simulink model "Final_Q2_j"  (R2019a)
settings: Solver=ode1  StartTime=0.0  StopTime=60  FixedStep=0.01  RelTol=1e-3  EnableMultiTasking=on
libraries: simulink x4
settings Model: Creator=enesu  LastModifiedBy=hp
settings SolverCC: AutoInsertRateTranBlk=on

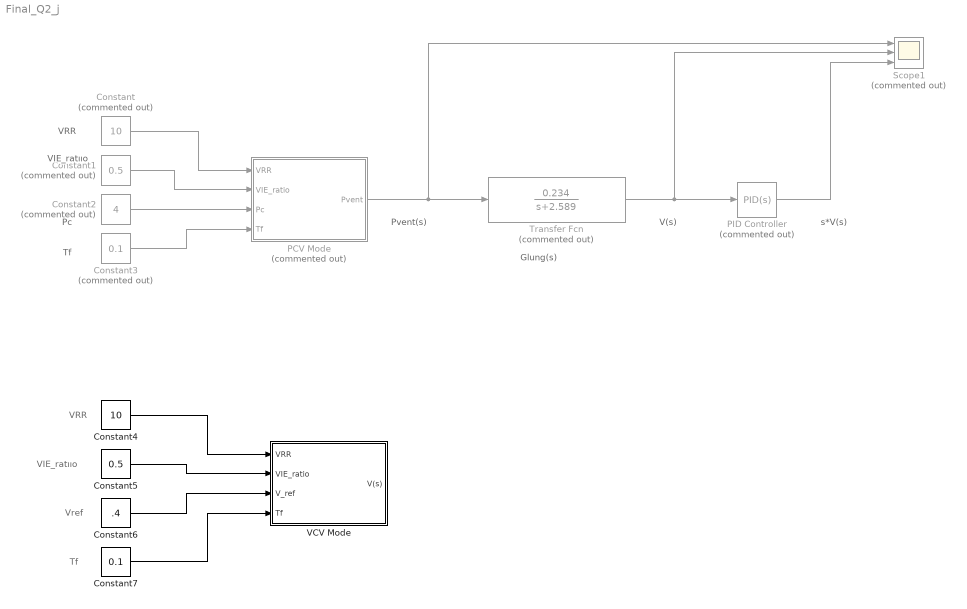
== system Final_Q2_j ==
  note: VIE_ratııo
  note: VRR
  note: Tf
  note: Vref
  note: VIE_ratııo
  note: VRR
  note: Pvent(s)
  note: Glung(s)
  note: s*V(s)
  note: V(s)
  note: Pc
  note: Tf
  Constant : Constant  Commented=on  Value=10  VectorParams1D=off
  Constant1 : Constant  Commented=on  Value=0.5
  Constant2 : Constant  Commented=on  Value=4
  Constant3 : Constant  Commented=on  Value=0.1
  Constant4 : Constant  Value=10
  Constant5 : Constant  Value=0.5
  Constant6 : Constant  Value=.4
  Constant7 : Constant  Value=0.1
  PCV Mode : Subsystem  Commented=on
  PID Controller : simulink/Continuous/PID Controller  Commented=on  Controller=PID  Form=Parallel  TimeDomain=Continuous-time  SampleTime=-1  IntegratorMethod=Forward Euler  FilterMethod=Forward Euler  ControllerParametersSource=internal  P=0  I=0  D=1  UseFilter=on  N=100  TunerSelectOption=Transfer Function Based (PID Tuner App)  InitialConditionSource=internal  InitialConditionForIntegrator=0  InitialConditionForFilter=0  DifferentiatorICPrevScaledInput=0  ExternalReset=none  TrackingMode=off  Kt=1  LimitOutput=off  UpperSaturationLimit=inf  LowerSaturationLimit=-inf  LinearizeAsGain=on  AntiWindupMode=none  Kb=1  POutMin=[]  POutMax=[]  IOutMin=[]  IOutMax=[]  DOutMin=[]  DOutMax=[]  NOutMin=[]  NOutMax=[]  SumOutMin=[]  SumOutMax=[]  SaturationOutMin=[]  SaturationOutMax=[]  PParamMin=[]  PParamMax=[]  IParamMin=[]  IParamMax=[]  DParamMin=[]  DParamMax=[]  NParamMin=[]  NParamMax=[]  KbParamMin=[]  KbParamMax=[]  KtParamMin=[]  KtParamMax=[]  KbOutMin=[]  KbOutMax=[]  KtOutMin=[]  KtOutMax=[]  IntegratorOutMin=[]  IntegratorOutMax=[]  FilterOutMin=[]  FilterOutMax=[]  SumI1OutMin=[]  SumI1OutMax=[]  SumI2OutMin=[]  SumI2OutMax=[]  SumI3OutMin=[]  SumI3OutMax=[]  SumI4OutMin=[]  SumI4OutMax=[]  SumDOutMin=[]  SumDOutMax=[]  DifferentiatorOutMin=[]  DifferentiatorOutMax=[]  FilterDiffOutCoefMin=[]  FilterDiffOutCoefMax=[]  ReciprocalOutMin=[]  ReciprocalOutMax=[]  SumDenOutMin=[]  SumDenOutMax=[]  SumNumOutMin=[]  SumNumOutMax=[]  DivideOutMin=[]  DivideOutMax=[]  IntegratorContinuousStateAttributes=''  IntegratorStateMustResolveToSignalObject=off  IntegratorRTWStateStorageClass=Auto  FilterContinuousStateAttributes=''  FilterStateMustResolveToSignalObject=off  FilterRTWStateStorageClass=Auto  ParallelPVariant=InternalParameters  IdealPVariant=Disabled  IVariant=InternalParameters  DVariant=InternalParameters  IntegratorVariant=Continuous  SatVariant=Disabled  AWVariant=Passthrough  PCopyVariant=Disabled  TRVariant=Disabled  FdbkBlocksVariant=Forward  IdealPFdbkVariant=Disabled  SatFdbkVariant=Disabled  DerivativeFilterVariant=ContFilter  NVariant=InternalParameters  NCopyVariant=Disabled  FilterICVariant=InternalICsFilter  IntegratorICVariant=InternalICs  ExternalResetVariant=Disabled  TRSumVariant=Passthrough  SumFdbkVariant=Disabled  SumVariant=Sum_PID
  Scope1 : Scope  Commented=on  NumInputPorts=3
  Transfer Fcn : TransferFcn  Commented=on  Numerator=[ 0.234 ]  Denominator=[1 2.589]
  VCV Mode : Subsystem
  wires:
  Constant/1 -> PCV Mode/1(VRR)
  Constant1/1 -> PCV Mode/2(VIE_ratio)
  Constant2/1 -> PCV Mode/3(Pc)
  Transfer Fcn/1 -> Scope1/2, PID Controller/1
  Constant3/1 -> PCV Mode/4(Tf)
  Constant6/1 -> VCV Mode/3(V_ref)
  Constant5/1 -> VCV Mode/2(VIE_ratio)
  Constant4/1 -> VCV Mode/1(VRR)
  PID Controller/1 -> Scope1/3
  Constant7/1 -> VCV Mode/4(Tf)
  PCV Mode/1(Pvent) -> Scope1/1, Transfer Fcn/1

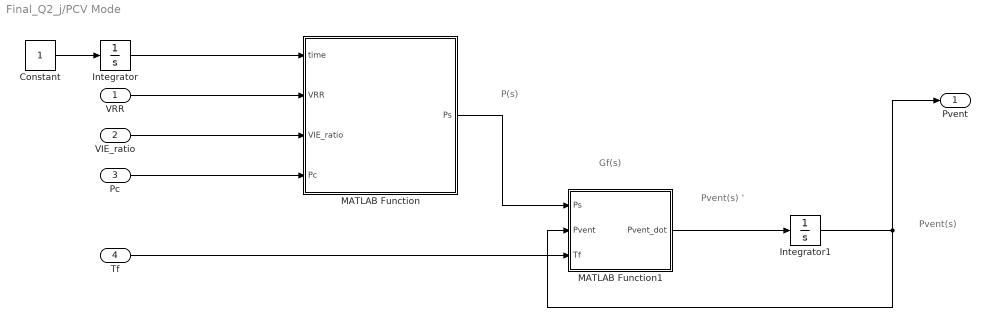
== system Final_Q2_j/PCV Mode ==
  note: P(s)
  note: Gf(s)
  note: Pvent(s) '
  note: Pvent(s)
  VRR : Inport
  VIE_ratio : Inport  Port=2
  Pc : Inport  Port=3
  Tf : Inport  Port=4
  Constant : Constant
  Integrator : Integrator
  Integrator1 : Integrator
  MATLAB Function : MATLAB Function  TreatAsAtomicUnit=on
  MATLAB Function1 : MATLAB Function  TreatAsAtomicUnit=on
  Pvent : Outport  VectorParamsAs1DForOutWhenUnconnected=on
  wires:
  Constant/1 -> Integrator/1
  Integrator/1 -> MATLAB Function/1(time)
  VRR/1 -> MATLAB Function/2(VRR)
  VIE_ratio/1 -> MATLAB Function/3(VIE_ratio)
  Pc/1 -> MATLAB Function/4(Pc)
  Tf/1 -> MATLAB Function1/3(Tf)
  MATLAB Function/1(Ps) -> MATLAB Function1/1(Ps)
  MATLAB Function1/1(Pvent_dot) -> Integrator1/1
  Integrator1/1 -> Pvent/1, MATLAB Function1/2(Pvent)

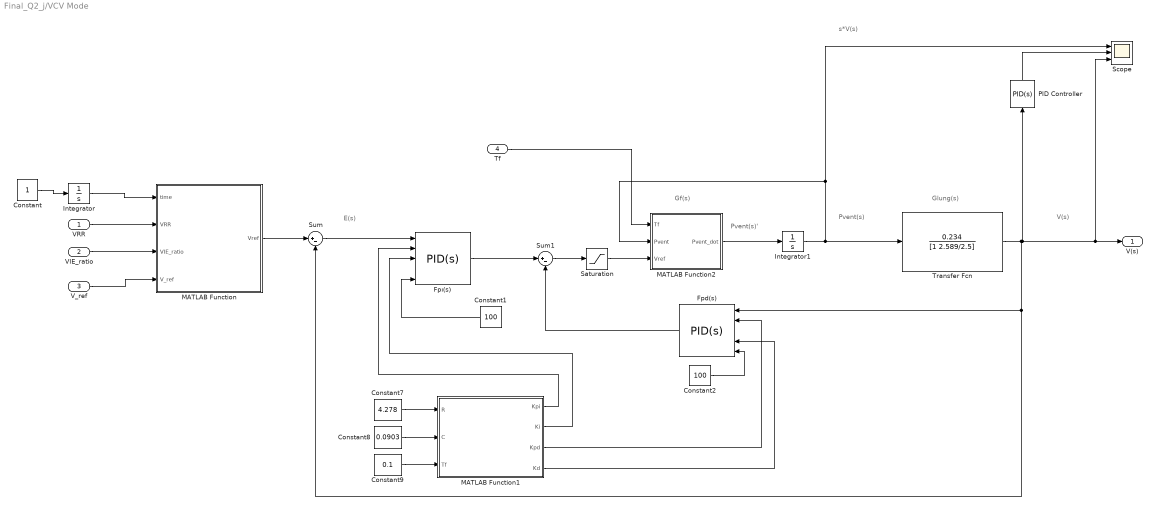
== system Final_Q2_j/VCV Mode ==
  note: Gf(s)
  note: Glung(s)
  note: s*V(s)
  note: V(s)
  note: Pvent(s)'
  note: Pvent(s)
  note: E(s)
  VRR : Inport
  VIE_ratio : Inport  Port=2
  V_ref : Inport  Port=3
  Tf : Inport  Port=4
  Constant : Constant
  Constant1 : Constant  Value=100
  Constant2 : Constant  Value=100
  Constant7 : Constant  Value=4.278
  Constant8 : Constant  Value=0.0903
  Constant9 : Constant  Value=0.1
  Fpd(s) : simulink/Continuous/PID Controller  Controller=PID  Form=Parallel  TimeDomain=Continuous-time  SampleTime=-1  IntegratorMethod=Forward Euler  FilterMethod=Forward Euler  ControllerParametersSource=external  P=1  I=1  D=0  UseFilter=on  N=100  TunerSelectOption=Transfer Function Based (PID Tuner App)  InitialConditionSource=internal  InitialConditionForIntegrator=0  InitialConditionForFilter=0  DifferentiatorICPrevScaledInput=0  ExternalReset=none  TrackingMode=off  Kt=1  LimitOutput=off  UpperSaturationLimit=115  LowerSaturationLimit=0  LinearizeAsGain=on  AntiWindupMode=none  Kb=1  POutMin=[]  POutMax=[]  IOutMin=[]  IOutMax=[]  DOutMin=[]  DOutMax=[]  NOutMin=[]  NOutMax=[]  SumOutMin=[]  SumOutMax=[]  SaturationOutMin=[]  SaturationOutMax=[]  PParamMin=[]  PParamMax=[]  IParamMin=[]  IParamMax=[]  DParamMin=[]  DParamMax=[]  NParamMin=[]  NParamMax=[]  KbParamMin=[]  KbParamMax=[]  KtParamMin=[]  KtParamMax=[]  KbOutMin=[]  KbOutMax=[]  KtOutMin=[]  KtOutMax=[]  IntegratorOutMin=[]  IntegratorOutMax=[]  FilterOutMin=[]  FilterOutMax=[]  SumI1OutMin=[]  SumI1OutMax=[]  SumI2OutMin=[]  SumI2OutMax=[]  SumI3OutMin=[]  SumI3OutMax=[]  SumI4OutMin=[]  SumI4OutMax=[]  SumDOutMin=[]  SumDOutMax=[]  DifferentiatorOutMin=[]  DifferentiatorOutMax=[]  FilterDiffOutCoefMin=[]  FilterDiffOutCoefMax=[]  ReciprocalOutMin=[]  ReciprocalOutMax=[]  SumDenOutMin=[]  SumDenOutMax=[]  SumNumOutMin=[]  SumNumOutMax=[]  DivideOutMin=[]  DivideOutMax=[]  IntegratorContinuousStateAttributes=''  IntegratorStateMustResolveToSignalObject=off  IntegratorRTWStateStorageClass=Auto  FilterContinuousStateAttributes=''  FilterStateMustResolveToSignalObject=off  FilterRTWStateStorageClass=Auto  ParallelPVariant=ExternalParameters  IdealPVariant=Disabled  IVariant=ExternalParameters  DVariant=ExternalParameters  IntegratorVariant=Continuous  SatVariant=Disabled  AWVariant=Passthrough  PCopyVariant=Disabled  TRVariant=Disabled  FdbkBlocksVariant=Forward  IdealPFdbkVariant=Disabled  SatFdbkVariant=Disabled  DerivativeFilterVariant=ContFilter  NVariant=ExternalParameters  NCopyVariant=Disabled  FilterICVariant=InternalICsFilter  IntegratorICVariant=InternalICs  ExternalResetVariant=Disabled  TRSumVariant=Passthrough  SumFdbkVariant=Disabled  SumVariant=Sum_PID
  Fpı(s) : simulink/Continuous/PID Controller  Controller=PID  Form=Parallel  TimeDomain=Continuous-time  SampleTime=-1  IntegratorMethod=Forward Euler  FilterMethod=Forward Euler  ControllerParametersSource=external  P=1  I=1  D=0  UseFilter=on  N=100  TunerSelectOption=Transfer Function Based (PID Tuner App)  InitialConditionSource=internal  InitialConditionForIntegrator=0  InitialConditionForFilter=0  DifferentiatorICPrevScaledInput=0  ExternalReset=none  TrackingMode=off  Kt=1  LimitOutput=off  UpperSaturationLimit=inf  LowerSaturationLimit=0  LinearizeAsGain=on  AntiWindupMode=none  Kb=1  POutMin=[]  POutMax=[]  IOutMin=[]  IOutMax=[]  DOutMin=[]  DOutMax=[]  NOutMin=[]  NOutMax=[]  SumOutMin=[]  SumOutMax=[]  SaturationOutMin=[]  SaturationOutMax=[]  PParamMin=[]  PParamMax=[]  IParamMin=[]  IParamMax=[]  DParamMin=[]  DParamMax=[]  NParamMin=[]  NParamMax=[]  KbParamMin=[]  KbParamMax=[]  KtParamMin=[]  KtParamMax=[]  KbOutMin=[]  KbOutMax=[]  KtOutMin=[]  KtOutMax=[]  IntegratorOutMin=[]  IntegratorOutMax=[]  FilterOutMin=[]  FilterOutMax=[]  SumI1OutMin=[]  SumI1OutMax=[]  SumI2OutMin=[]  SumI2OutMax=[]  SumI3OutMin=[]  SumI3OutMax=[]  SumI4OutMin=[]  SumI4OutMax=[]  SumDOutMin=[]  SumDOutMax=[]  DifferentiatorOutMin=[]  DifferentiatorOutMax=[]  FilterDiffOutCoefMin=[]  FilterDiffOutCoefMax=[]  ReciprocalOutMin=[]  ReciprocalOutMax=[]  SumDenOutMin=[]  SumDenOutMax=[]  SumNumOutMin=[]  SumNumOutMax=[]  DivideOutMin=[]  DivideOutMax=[]  IntegratorContinuousStateAttributes=''  IntegratorStateMustResolveToSignalObject=off  IntegratorRTWStateStorageClass=Auto  FilterContinuousStateAttributes=''  FilterStateMustResolveToSignalObject=off  FilterRTWStateStorageClass=Auto  ParallelPVariant=ExternalParameters  IdealPVariant=Disabled  IVariant=ExternalParameters  DVariant=ExternalParameters  IntegratorVariant=Continuous  SatVariant=Disabled  AWVariant=Passthrough  PCopyVariant=Disabled  TRVariant=Disabled  FdbkBlocksVariant=Forward  IdealPFdbkVariant=Disabled  SatFdbkVariant=Disabled  DerivativeFilterVariant=ContFilter  NVariant=ExternalParameters  NCopyVariant=Disabled  FilterICVariant=InternalICsFilter  IntegratorICVariant=InternalICs  ExternalResetVariant=Disabled  TRSumVariant=Passthrough  SumFdbkVariant=Disabled  SumVariant=Sum_PID
  Integrator : Integrator
  Integrator1 : Integrator
  MATLAB Function : MATLAB Function  TreatAsAtomicUnit=on
  MATLAB Function1 : MATLAB Function  TreatAsAtomicUnit=on
  MATLAB Function2 : MATLAB Function  TreatAsAtomicUnit=on
  PID Controller : simulink/Continuous/PID Controller  Controller=PID  Form=Parallel  TimeDomain=Continuous-time  SampleTime=-1  IntegratorMethod=Forward Euler  FilterMethod=Forward Euler  ControllerParametersSource=internal  P=0  I=0  D=1  UseFilter=on  N=100  TunerSelectOption=Transfer Function Based (PID Tuner App)  InitialConditionSource=internal  InitialConditionForIntegrator=0  InitialConditionForFilter=0  DifferentiatorICPrevScaledInput=0  ExternalReset=none  TrackingMode=off  Kt=1  LimitOutput=off  UpperSaturationLimit=inf  LowerSaturationLimit=-inf  LinearizeAsGain=on  AntiWindupMode=none  Kb=1  POutMin=[]  POutMax=[]  IOutMin=[]  IOutMax=[]  DOutMin=[]  DOutMax=[]  NOutMin=[]  NOutMax=[]  SumOutMin=[]  SumOutMax=[]  SaturationOutMin=[]  SaturationOutMax=[]  PParamMin=[]  PParamMax=[]  IParamMin=[]  IParamMax=[]  DParamMin=[]  DParamMax=[]  NParamMin=[]  NParamMax=[]  KbParamMin=[]  KbParamMax=[]  KtParamMin=[]  KtParamMax=[]  KbOutMin=[]  KbOutMax=[]  KtOutMin=[]  KtOutMax=[]  IntegratorOutMin=[]  IntegratorOutMax=[]  FilterOutMin=[]  FilterOutMax=[]  SumI1OutMin=[]  SumI1OutMax=[]  SumI2OutMin=[]  SumI2OutMax=[]  SumI3OutMin=[]  SumI3OutMax=[]  SumI4OutMin=[]  SumI4OutMax=[]  SumDOutMin=[]  SumDOutMax=[]  DifferentiatorOutMin=[]  DifferentiatorOutMax=[]  FilterDiffOutCoefMin=[]  FilterDiffOutCoefMax=[]  ReciprocalOutMin=[]  ReciprocalOutMax=[]  SumDenOutMin=[]  SumDenOutMax=[]  SumNumOutMin=[]  SumNumOutMax=[]  DivideOutMin=[]  DivideOutMax=[]  IntegratorContinuousStateAttributes=''  IntegratorStateMustResolveToSignalObject=off  IntegratorRTWStateStorageClass=Auto  FilterContinuousStateAttributes=''  FilterStateMustResolveToSignalObject=off  FilterRTWStateStorageClass=Auto  ParallelPVariant=InternalParameters  IdealPVariant=Disabled  IVariant=InternalParameters  DVariant=InternalParameters  IntegratorVariant=Continuous  SatVariant=Disabled  AWVariant=Passthrough  PCopyVariant=Disabled  TRVariant=Disabled  FdbkBlocksVariant=Forward  IdealPFdbkVariant=Disabled  SatFdbkVariant=Disabled  DerivativeFilterVariant=ContFilter  NVariant=InternalParameters  NCopyVariant=Disabled  FilterICVariant=InternalICsFilter  IntegratorICVariant=InternalICs  ExternalResetVariant=Disabled  TRSumVariant=Passthrough  SumFdbkVariant=Disabled  SumVariant=Sum_PID
  Saturation : Saturate  UpperLimit=30  LowerLimit=0
  Scope : Scope  NumInputPorts=3
  Sum : Sum  Inputs=|+-
  Sum1 : Sum  Inputs=|+-
  Transfer Fcn : TransferFcn  Numerator=[0.234]  Denominator=[1 2.589/2.5]
  V(s) : Outport  VectorParamsAs1DForOutWhenUnconnected=on
  wires:
  Constant/1 -> Integrator/1
  Integrator/1 -> MATLAB Function/1(time)
  VRR/1 -> MATLAB Function/2(VRR)
  VIE_ratio/1 -> MATLAB Function/3(VIE_ratio)
  V_ref/1 -> MATLAB Function/4(V_ref)
  Constant7/1 -> MATLAB Function1/1(R)
  MATLAB Function1/4(Kd) -> Fpd(s)/4
  Constant9/1 -> MATLAB Function1/3(Tf)
  Constant8/1 -> MATLAB Function1/2(C)
  Sum/1 -> Fpı(s)/1
  Fpı(s)/1 -> Sum1/1
  MATLAB Function1/1(Kpi) -> Fpı(s)/2
  MATLAB Function1/2(Ki) -> Fpı(s)/3
  MATLAB Function1/3(Kpd) -> Fpd(s)/2
  Integrator1/1 -> Transfer Fcn/1, Scope/1, MATLAB Function2/2(Pvent)
  MATLAB Function2/1(Pvent_dot) -> Integrator1/1
  Transfer Fcn/1 -> PID Controller/1, V(s)/1, Scope/3, Sum/2, Fpd(s)/1
  Constant1/1 -> Fpı(s)/5
  Constant2/1 -> Fpd(s)/5
  Fpd(s)/1 -> Sum1/2
  Sum1/1 -> Saturation/1
  PID Controller/1 -> Scope/2
  Tf/1 -> MATLAB Function2/1(Tf)
  Saturation/1 -> MATLAB Function2/3(Vref)
  MATLAB Function/1(Vref) -> Sum/1

== matlab function Final_Q2_j/VCV Mode/MATLAB Function ==
  data: time input; Vref output; VRR input; VIE_ratio input; V_ref input
function Vref = Vref_producer(time,VRR,VIE_ratio ,V_ref)

stop_time = 60; % stop time is given as 60 seconds

% Ti - Inspiratory Time (s)     Te - Expiratory Time (s)
% VRR - Ventilator Respiratory Rate (breaths/min) is 10.
% VIE_ratio ventilator inspiratory/expiratory rate is 0.5.
% 
% There are 2 two equations.
%
%   60
% ------ = Ti + Te     and     Ti = Te x VIE_ratio
%   VRR
% 
% in matrix form;
%  _  _     _             _     _  _
% | 60 |   | 1      1      |   | Ti |
% | 0  | = | 1  -VIE_ratio | * | Te |
%  -  -     -             -     -  -
%
%   b = A.T 
%   T = inv(A).b

A = [ 1 1 ; 1 -VIE_ratio];
B = [stop_time/VRR ; 0];

T = inv(A)*B;

Ti = T(1); % Ti
Te = T(2); % Te



% We can set the period duration of the desired square wave 
% as [0, Ti + Te] by performing modulus operation.
time = mod(time , Ti + Te ); 

if( time <= Ti)
    Vref = V_ref; 
else
    Vref = 0; 
end
end

== matlab function Final_Q2_j/PCV Mode/MATLAB Function ==
  data: time input; Ps output; VRR input; VIE_ratio input; Pc input
function Ps = P_producer(time,VRR,VIE_ratio ,Pc)

stop_time = 60; % stop time is given as 60 seconds

% Ti - Inspiratory Time (s)     Te - Expiratory Time (s)
% VRR - Ventilator Respiratory Rate (breaths/min) is 10.
% VIE_ratio ventilator inspiratory/expiratory rate is 0.5.
% 
% There are 2 two equations.
%
%   60
% ------ = Ti + Te     and     Ti = Te x VIE
%   VRR
% 
% in matrix form;
%  _  _     _             _     _  _
% | 60 |   | 1      1      |   | Ti |
% | 0  | = | 1  -VIE_ratio | * | Te |
%  -  -     -             -     -  -
%
%   b = A.T 
%   T = inv(A).b

A = [ 1 1 ; 1 -VIE_ratio];
B = [stop_time/VRR ; 0];

T = inv(A)*B;

Ti = T(1); % Ti
Te = T(2); % Te



% We can set the period duration of the desired square wave 
% as [0, Ti + Te] by performing modulus operation.
time = mod(time , Ti + Te ); 

if( time <= Ti)
    Ps = Pc; 
else
    Ps = 0; 
end
end

== matlab function Final_Q2_j/VCV Mode/MATLAB Function1 ==
  data: R input; Kpi output; Ki output; C input; Tf input; Kpd output; Kd output
function [Kpi,Ki, Kpd ,Kd ] = calcute_control_param(R,C,Tf)
Kpi = (16*R)/(25*Tf);
Kpd = (32*R)/(5*Tf) - 1/C;
Ki = (64*R)/(25*Tf^2);
Kd = (23*R)/5 - Tf/C;
end

== matlab function Final_Q2_j/PCV Mode/MATLAB Function1 ==
  data: Ps input; Pvent_dot output; Pvent input; Tf input
function Pvent_dot = filter(Ps,Pvent,Tf)
% Gf(s) = Pvent/ Ps = 1/( Tf*s + 1)
% Pvent* (Tf*s + 1) = Ps
% Pvent*Tf*s + Pvent = Ps
%
% In time domain 
% Pvent(t)' * Tf + Pvent(t) = P(t)
% Pvent(t)' = (P(t)  - Pvent(t))/ Tf
Pvent_dot = (Ps  - Pvent)/ Tf;

end

== matlab function Final_Q2_j/VCV Mode/MATLAB Function2 ==
  data: Tf input; Pvent input; Vref input; Pvent_dot output
function Pvent_dot = filter(Tf,Pvent,Vref)
% Gf(s) = Pvent/ Vref = 1/( Tf*s + 1)
% Pvent* (Tf*s + 1) = Vref
% Pvent*Tf*s + Pvent = Vref
%
% In time domain 
% Pvent(t)' * Tf + V(t) = Vref(t)
% Pvent(t)' = (Vref(t)  - Pvent(t))/ Tf
% Pvent_dot = (Vref  - Pvent)/ Tf;
Pvent_dot = (Vref  - Pvent)/ Tf;

end
